simulink model "onlab_2"  (R2024b)
settings: Solver=VariableStepAuto  StartTime=0.0  StopTime=16  RelTol=1e-3
libraries: simulink x2
settings Model: Creator=Asus  LastModifiedBy=Asus

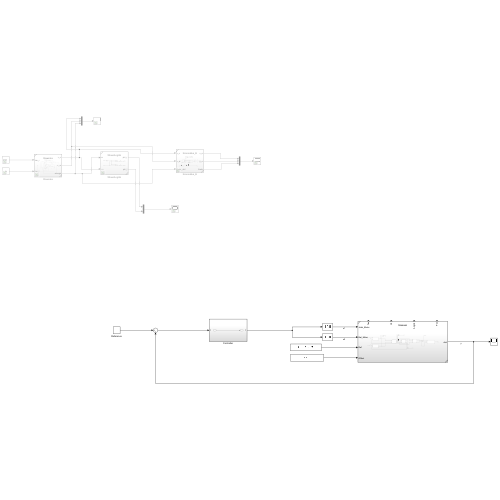
[thumbnail: Simulink's stored preview of the top-level diagram]
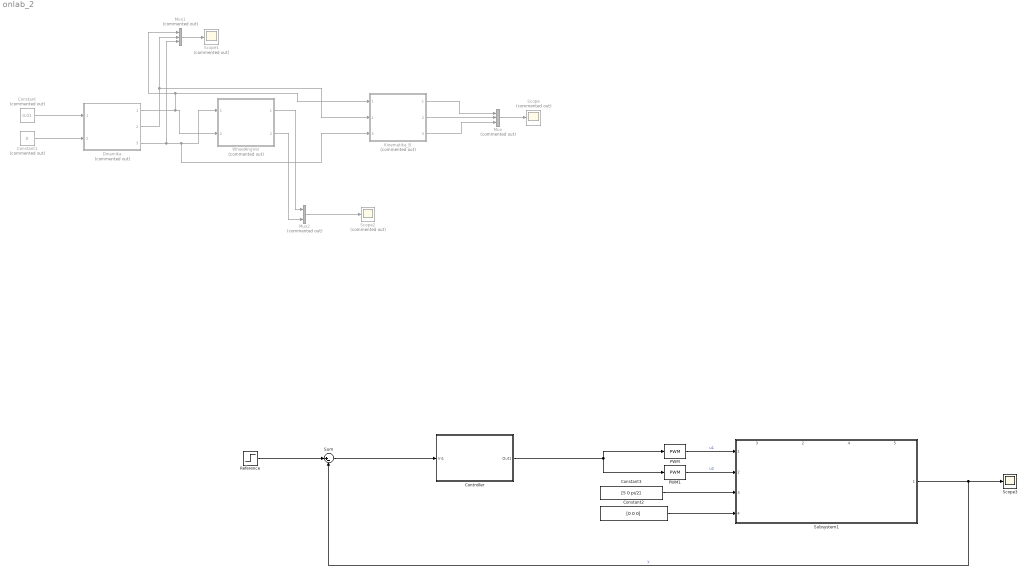
== system onlab_2 ==
  Constant : Constant  Commented=on  Value=0.01
  Constant1 : Constant  Commented=on  Value=0
  Constant2 : Constant  Value=[0 0 0]
  Constant3 : Constant  Value=[5 0 pi/2]
  Controller : Subsystem
  Dinamika : Subsystem  Commented=on  ReferencedSubsystem=Dinamika
  Kinematika_B : Subsystem  Commented=on  ReferencedSubsystem=Kinematika_B
  Mux : Mux  Commented=on  Inputs=3
  Mux1 : Mux  Commented=on  Inputs=3
  Mux2 : Mux  Commented=on  Inputs=2
  PWM : simulink/Discontinuities/PWM  DisableCoverage=on  Period=1  InitialDelay=0  DisallowZeroDutyCycle=off  RunAtFixedTimeIntervals=off  SampleTime=0.1
  PWM1 : simulink/Discontinuities/PWM  DisableCoverage=on  Period=1  InitialDelay=0  DisallowZeroDutyCycle=off  RunAtFixedTimeIntervals=off  SampleTime=0.1
  Reference : Step  Time=0.5  After=-6  SampleTime=0
  Scope : Scope  Commented=on
  Scope1 : Scope  Commented=on
  Scope2 : Scope  Commented=on
  Scope3 : Scope
  Subsystem1 : Subsystem  ReferencedSubsystem=Szakasz
      settings: PortSchema="{\"entries\":[{\"content\":{\"sides\":[{\"content\":{\"connectorIds\":[\"In1\",\"In2\",\"In3\",\"In4\"]},\"type\":\"ConnectorPlacement.EquallySpacedRectSide\",\"uuid\":\"a36feab4-e4f6-449b-af94-39429bfcb95e\"},{\"content\":{\"connectorIds\":[\"Out1\"],\"side\":\"RIGHT\"},\"type\":\"ConnectorPlacement.EquallySpacedRectSide\",\"uuid\":\"02fb0c92-7c86-43ad-8702-b2facecb5ebc\"},{\"content\":{\"connectorIds\":[\"Out3\",\"Out2\",\"Out4\",\"Out5\"],\"side\":\"TOP\"},\"type\":\"ConnectorPlacement.EquallySpacedRectSide\",\"uuid\":\"1b9f3d57-250f-49eb-babd-b9abb8485c57\"}]},\"type\":\"ConnectorPlacement.EquallySpacedConnector\",\"uuid\":\"c1e7b1f3-c6dd-46bd-a9ee-6c337d0ecb94\"}],\"packageUris\":[\"http://schema.mathworks.com/mf0/Connector/R2020b\"],\"version\":\"1.0\"}"
  Sum : Sum  Inputs=|+-
  WheelAngVel : Subsystem  Commented=on  ReferencedSubsystem=WheelAngVel
  wires:
  Dinamika/1 -> Mux1/1, Kinematika_B/1, WheelAngVel/2
  Dinamika/3 -> Mux1/3, Kinematika_B/3, WheelAngVel/1
  Dinamika/2 -> Kinematika_B/2, Mux1/2
  Kinematika_B/1 -> Mux/1
  Kinematika_B/2 -> Mux/2
  Kinematika_B/3 -> Mux/3
  Mux/1 -> Scope/1
  Mux1/1 -> Scope1/1
  WheelAngVel/2 -> Mux2/2
  Mux2/1 -> Scope2/1
  WheelAngVel/1 -> Mux2/1
  Constant/1 -> Dinamika/1
  Constant1/1 -> Dinamika/2
  PWM/1 -> Subsystem1/1  "u1"
  PWM1/1 -> Subsystem1/2  "u2"
  Constant2/1 -> Subsystem1/4
  Constant3/1 -> Subsystem1/3
  Controller/1(Out1) -> PWM/1, PWM1/1
  Subsystem1/1 -> Sum/2, Scope3/1  "y"
  Sum/1 -> Controller/1(In1)
  Reference/1 -> Sum/1

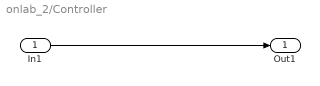
== system onlab_2/Controller ==
  In1 : Inport
  Out1 : Outport
  wires:
  In1/1 -> Out1/1
